simulink model "W04_5_offline"  (R2024b)
settings: Solver=ode4  StartTime=0.0  StopTime=80  FixedStep=0.05  RelTol=1e-3
values from neighbouring files (symbols this model uses):
  animate = 1    [W04_setup.m]
  tau_m = 0.30    (= 0.3)    [W04_setup.m]
settings Model: Creator=admin  LastModifiedBy=admin

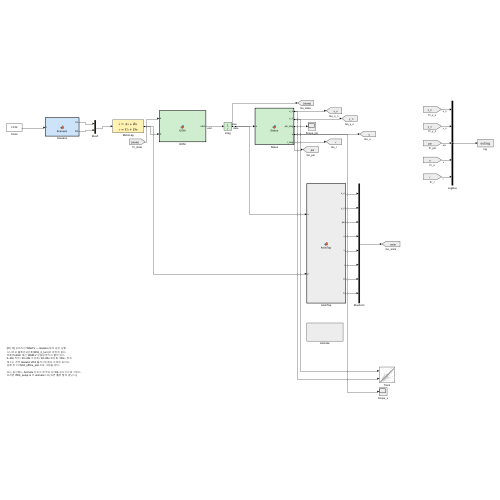
[thumbnail: Simulink's stored preview of the top-level diagram]
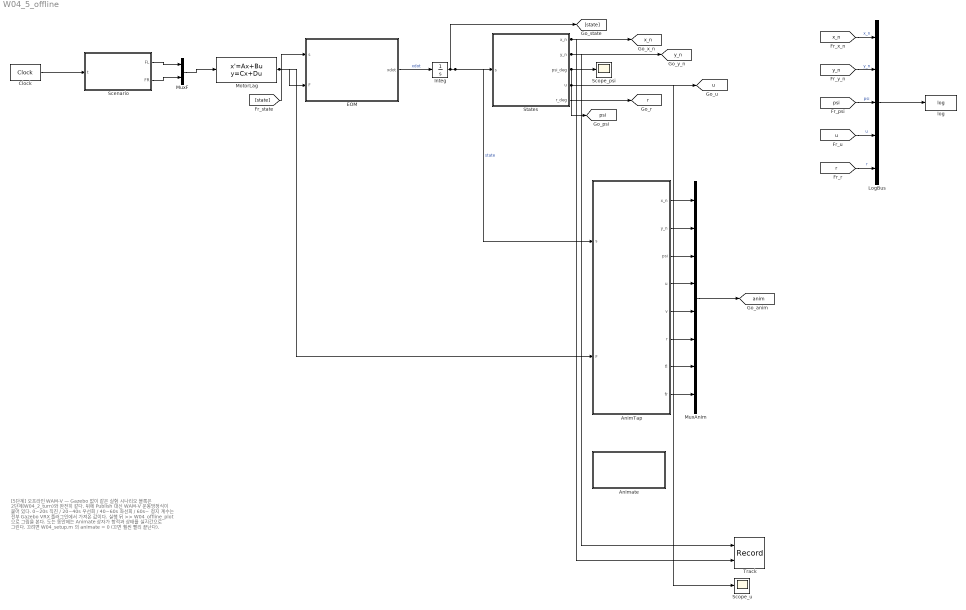
== system W04_5_offline ==
  note: [5단계] 오프라인 WAM-V — Gazebo 없이 같은 실험
      | 시나리오 블록은 2단계(W04_2_turn)와 완전히 같다.
      | 뒤에 Publish 대신 WAM-V 운동방정식이 붙어 있다.
      | 0~20s 직진 / 20~40s 우선회 / 40~60s 좌선회 / 60s~ 정지
      | 계수는 전부 Gazebo VRX 플러그인에서 가져온 값이다.
      | 실행 뒤 >> W04_offline_plot 으로 그림을 본다.
      |
      | 도는 동안에는 Animate 상자가 항적과 상태를 실시간으로 그린다.
      | 끄려면 W04_setup.m 의 animate = 0 (끄면 훨씬 빨리 끝난다).
  AnimTap : MATLAB Function  TreatAsAtomicUnit=on
  Animate : Subsystem
  Clock : DigitalClock  SampleTime=0.05
  EOM : MATLAB Function  TreatAsAtomicUnit=on
  Integ : Integrator  InitialCondition=[0;0;0;0;0;0]
  LogBus : BusCreator  Inputs=5
  MotorLag : StateSpace  A=-eye(2)/tau_m  B=eye(2)/tau_m  C=eye(2)  D=zeros(2)  InitialCondition=zeros(2,1)
  MuxAnim : Mux  Inputs=8
  MuxF : Mux  Inputs=2
  Scenario : MATLAB Function  TreatAsAtomicUnit=on
  Scope_psi : Scope
  Scope_u : Scope
  States : MATLAB Function  TreatAsAtomicUnit=on
  Track : Record  FileSettingsInternal="{\"entries\":[{\"content\":{\"excelSettings\":{\"content\":{},\"type\":\"Streamout.ExcelSettings\"}},\"type\":\"Streamout.FileSettingStorage\",\"uuid\":\"\"}],\"packageUris\":[\"http:\\/\\/schema.mathworks.com\\/mf0\\/streamout_blocks\\/R2020a\"],\"version\":\"1.0\"}"  Layout=[1 1]  SignalsInternal="{\"entries\":[{\"content\":{\"signals\":[{\"content\":{\"blockPath\":[],\"dimensions\":[1],\"domain\":\"\",\"lineColor\":\"#a2142f\",\"plots\":[ 1 ],\"port\":1,\"signalID\":1,\"signalName\":\"XY Graph:1\"},\"type\":\"RecordBlkView.Signal\",\"uuid\":\"\"},{\"content\":{\"blockPath\":[],\"dimensions\":[1],\"domain\":\"\",\"lineColor\":\"#139fff\",\"plots\":[ 1 ],\"port\":2,\"signalID\":2,\"signalName\":\"XY Graph:2\"},\"type\":\"RecordBlkView.Signal\",\"uuid\":\"\"}]},\"type\":\"RecordBlkView.InputSignals\",\"uuid\":\"\"}],\"packageUris\":[\"http:\\/\\/schema.mathworks.com\\/mf0\\/streamout_blocks\\/R2020a\"],\"version\":\"1.0\"}"  VisualizationBindings="{\"xyplotplugin\":{\"info\":[{\"series\":[{\"bindingParametersList\":[{\"parameter\":\"X-Axis\",\"signalID\":1,\"signalName\":\"XY Graph:1\"},{\"parameter\":\"Y-Axis\",\"signalID\":2,\"signalName\":\"XY Graph:2\"}],\"seriesID\":0}],\"subplotID\":1}]}}"  CompatibilityTag=XY
  log : ToWorkspace  VariableName=log  SaveFormat=Timeseries  SampleTime=0.05
  tag scope: anim=global, psi=global, r=global, u=global, x_n=global, y_n=global
  wires:
  Clock/1 -> Scenario/1(t)
  Scenario/1(FL) -> MuxF/1
  Scenario/2(FR) -> MuxF/2
  MuxF/1 -> MotorLag/1
  MotorLag/1 -> EOM/2(F), AnimTap/2(F)
  EOM/1(xdot) -> Integ/1  "xdot"
  Integ/1 -> States/1(s), AnimTap/1(s), [state]  "state"
  States/4(u) -> Scope_u/1, [u]
  States/3(psi_deg) -> Scope_psi/1, [psi]
  States/5(r_deg) -> [r]
  [x_n] -> LogBus/1  "x_n"
  [y_n] -> LogBus/2  "y_n"
  [psi] -> LogBus/3  "psi"
  [u] -> LogBus/4  "u"
  [r] -> LogBus/5  "r"
  LogBus/1 -> log/1
  AnimTap/1(x_n) -> MuxAnim/1
  AnimTap/2(y_n) -> MuxAnim/2
  AnimTap/3(psi) -> MuxAnim/3
  AnimTap/4(u) -> MuxAnim/4
  AnimTap/5(v) -> MuxAnim/5
  AnimTap/6(r) -> MuxAnim/6
  AnimTap/7(fl) -> MuxAnim/7
  AnimTap/8(fr) -> MuxAnim/8
  MuxAnim/1 -> [anim]
  States/1(x_n) -> [x_n], Track/2
  States/2(y_n) -> [y_n], Track/1
  [state] -> EOM/1(s)

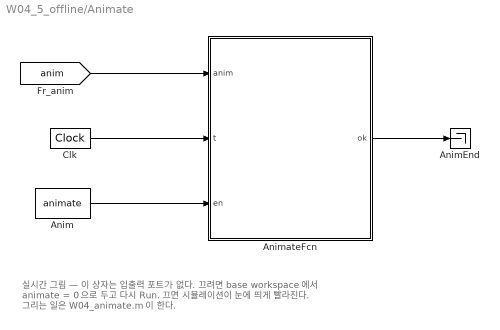
== system W04_5_offline/Animate ==
  note: 실시간 그림 — 이 상자는 입출력 포트가 없다.
      | 끄려면 base workspace 에서  animate = 0  으로 두고 다시 Run.
      | 끄면 시뮬레이션이 눈에 띄게 빨라진다.
      | 그리는 일은 W04_animate.m 이 한다.
  Anim : Constant  Value=animate
  AnimEnd : Terminator
  AnimateFcn : MATLAB Function  TreatAsAtomicUnit=on
  Clk : DigitalClock  SampleTime=0.05
  wires:
  [anim] -> AnimateFcn/1(anim)
  Clk/1 -> AnimateFcn/2(t)
  Anim/1 -> AnimateFcn/3(en)
  AnimateFcn/1(ok) -> AnimEnd/1

== matlab function W04_5_offline/EOM ==
  data: s input; xdot output; F input
function xdot = EOM(s, F)
%#codegen
% 3-DOF WAM-V equations of motion in NED.
% Every coefficient below is taken from the Gazebo VRX plugins, so
% this model and the simulator answer the same question the same way.
%   drag : wamv_gazebo_dynamics_plugin.xacro (SimpleHydrodynamics)
%   mass : 211 kg = 180 hull + 2x15 engines + 2x0.5 propellers
%   added mass is zero in VRX (xDotU = yDotV = nDotR = 0)
%   s = [u v r x_n y_n psi]    F = [FL; FR]

mm  = 211;    Izz = 653;
Xu  = 100;    Xuu = 150;
Yv  = 100;    Yvv = 100;
Nr  = 800;    Nrr = 800;
b   = 1.027135;          % half beam of the aft thrusters [m]

u = s(1); v = s(2); r = s(3); psi = s(6);

% differential thrust -> surge force and yaw moment
X = F(1) + F(2);
N = (F(1) - F(2))*b;

Dx = (Xu + Xuu*abs(u))*u;
Dy = (Yv + Yvv*abs(v))*v;
Dn = (Nr + Nrr*abs(r))*r;

du = (X - Dx)/mm + v*r;     % rigid-body Coriolis
dv = (  - Dy)/mm - u*r;
dr = (N - Dn)/Izz;

xdot = [du; dv; dr;
        u*cos(psi) - v*sin(psi);
        u*sin(psi) + v*cos(psi);
        r];

== matlab function W04_5_offline/Scenario ==
  data: t input; FL output; FR output
function [FL, FR] = Scenario(t)
%#codegen
% Time-based thrust scenario [N] - identical to W04_2_turn
if t < 20
    FL = 200;  FR = 200;   % go straight
elseif t < 40
    FL = 300;  FR =  50;   % turn starboard (right)
elseif t < 60
    FL =  50;  FR = 300;   % turn port (left)
else
    FL = 0;    FR = 0;     % stop
end

== matlab function W04_5_offline/States ==
  data: s input; x_n output; y_n output; psi_deg output; u output; r_deg output
function [x_n, y_n, psi_deg, u, r_deg] = States(s)
%#codegen
% Pull the numbers we want to look at out of the state.
x_n = s(4);
y_n = s(5);
psi_deg = s(6)*180/pi;
u  = s(1);
r_deg = s(3)*180/pi;

== matlab function W04_5_offline/AnimTap ==
  data: s input; x_n output; F input; y_n output; psi output; u output; v output; r output; fl output; fr output
function [x_n, y_n, psi, u, v, r, fl, fr] = AnimTap(s, F)
%#codegen
% Display-only tap. s = [u v r x_n y_n psi]', F = [FL; FR] after the
% motor lag, i.e. the thrust the hull actually feels.
x_n = s(4);
y_n = s(5);
psi = atan2(sin(s(6)), cos(s(6)));   % wrap to [-pi, pi]
u   = s(1);
v   = s(2);
r   = s(3);
fl  = F(1);
fr  = F(2);

== matlab function W04_5_offline/Animate/AnimateFcn ==
  data: anim input; ok output; t input; en input
function ok = AnimateFcn(anim, t, en)
%#codegen
% 실시간 그림. MATLAB Function 블록은 그림을 그리지 못하므로 그리는 함수를
% extrinsic 으로 선언한다 — 코드를 만들지 않고 평범한 MATLAB 을 부른다.
% en = base workspace 의 animate (0 이면 그리지 않는다).
%
% anim 은 Mux 로 묶어 온 여덟 신호다 (빌더의 animBundle 과 같은 순서).
%   1 x_n   2 y_n   3 psi   4 u   5 v   6 r   7 FL   8 FR
coder.extrinsic('W04_animate');
ok = 1;
if en > 0.5
    W04_animate(anim(1), anim(2), anim(3), anim(4), anim(5), anim(6), anim(7), anim(8), NaN, NaN, t);
end
